simulink model "B2B_MMC"  (R2018b)
settings: Solver=ode8  StartTime=0.0  StopTime=inf  FixedStep=10e-5  RelTol=1e-3
InitFcn:
  | Cd=100e-6;
  | Csm=3.3e-3;
  | L=4e-3;
  | R=0.1;
  | m=1;
  | N=9;
  | Nminus=N-1;
  | 
  | 
  | grid.vll_rms=10e3;
  | grid.f=50;
  | w=2*pi*grid.f;
  | grid.phase=0;
  | grid.va_peak=sqrt(2/3)*grid.vll_rms;
  | 
  | vd_ref=1.05*2*sqrt(2/3)*grid.vll_rms/m; % dc link voltage in pu
  | vsp_max=0.5*m*vd_ref; %phase voltage at phi=0
  | is_max=907;
  | Smax=3*grid.va_peak*is_max/2;
  | 
  | 
  | SCR= 100;  % INPUT SCR of grid at PCC = Ssc_grid/S_rated
  | %Calculated Grid impedance parameters
  | grid.L=grid.va_peak/(w*SCR*is_max); %Calculate Lg out of SRC and neglecting Rg
  | grid.R= w*grid.L/10;        % assume Rg = 10% of Xg [ohm];
  | grid.enable=1;
  | 
  | 
  | 
  | mmc1.load_percent=100;
  | mmc1.load_pf=0.9;
  | 
  | mmc2.load_percent=100;
  | mmc2.load_pf=0.9;
  | 
  | 
  | 
  | mmc1.occ_alpha = 2000;      % INPUT Desired BW output control test converter [rad/s]
  | mmc1.occ_alpha1 = 50;       % INPUT Desired BW of the resonant integrator [rad/s]
  | mmc1.occ_alpha_f = 1000;       % INPUT Desire BW of the VFF [rad/s]
  | 
  | mmc2.occ_alpha = 2000;      % INPUT Desired BW output control test converter [rad/s]
  | mmc2.occ_alpha1 = 50;       % INPUT Desired BW of the resonant integrator [rad/s}
  | mmc2.occ_alpha_f = 1000;       % INPUT Desire BW of the VFF [rad/s
  | 
  | 
  | mmc1.ccc_enable= 1; %INPUT enable ic controller
  | mmc1.ccc_time_enable= 0; %time when circ current control kicks in [s]
  | mmc1.ccc_alpha_cr= 30;  % INPUT BW of LPF for circ current to get the reference (dc value)[rad/s]
  | mmc1.ccc_Ra        = 10;       % INPUT Proportional gain of circ current control (R << Ra < Kp)
  | mmc1.ccc_alpha2 = 200;      % INPUT BW for circulating current test converter  (alpha_c < wgrid)[rad/s]
  | 
  | mmc2.ccc_enable= 1; %INPUT enable ic controller
  | mmc2.ccc_time_enable= 0; %time when circ current control kicks in [s]
  | mmc2.ccc_alpha_cr= 30;  % INPUT BW of LPF for circ current to get the reference (dc value)[rad/s]
  | mmc2.ccc_Ra        = 10;       % INPUT Proportional gain of circ current control (R << Ra < Kp)
  | mmc2.ccc_alpha2 = 200;      % INPUT BW for circulating current test converter  (alpha_c < wgrid)[rad/s]
  | 
  | 
  | mmc1.aec_enable_W= 1; %INPUT enable arm energy controller (Wsum and Wdelta)) at time_W_ctrl
  | ... (+31 lines)
libraries: powerlib x90, powerlib_meascontrol x10, rtlab x1, rtio_opalrt_op5142ex1 x1
(part 2 of 3)

== system B2B_MMC/SM_MMC/MMC1/convertor legs/lower arm a ==
  nla : Inport
  ila : Inport  Port=2
  Controlled Voltage Source : powerlib/Electrical Sources/Controlled Voltage Source  Initialize=on  Source_Type=AC  Amplitude=0  Phase=0  Frequency=0  Measurements=None
  Delay : Delay  DelayLength=1  InitialCondition=0
  Delay1 : Delay  DelayLength=1  InitialCondition=0
  Product : Product
  Product1 : Product
  Voltage Measurement : powerlib/Measurements/Voltage Measurement  PhasorSimulation=off  OutputType=Complex  PSBequivalent=0
  carm : powerlib/Elements/Series RLC Branch  LConnTagsString=__new0  RConnTagsString=__new0  BranchType=C  Resistance=1  Inductance=1e-3  SetiL0=off  InitialCurrent=0  Capacitance=Csm/N  Setx0=on  InitialVoltage=vd_ref  Measurements=None
  icap : powerlib/Electrical Sources/Controlled Current Source  Initialize=on  Source_Type=AC  Amplitude=0  Phase=0  Frequency=0  Measurements=None
  B : PMIOPort  Side=Left
  A : PMIOPort  Port=2  Side=Right
  vc_la : Outport
  wires:
  nla/1 -> Delay/1
  Product/1 -> Controlled Voltage Source/1
  ila/1 -> Delay1/1
  Delay/1 -> Product1/1, Product/2
  Product1/1 -> icap/1
  Voltage Measurement/1 -> vc_la/1, Product/1
  Delay1/1 -> Product1/2
  connections:
  Controlled Voltage Source/LConn1 -- B/RConn1
  Controlled Voltage Source/RConn1 -- A/RConn1
  Voltage Measurement/LConn1 -- carm/LConn1 -- icap/RConn1
  icap/LConn1 -- carm/RConn1 -- Voltage Measurement/LConn2

== system B2B_MMC/SM_MMC/MMC1/convertor legs/lower arm b ==
  nlb : Inport
  ilb : Inport  Port=2
  Controlled Voltage Source : powerlib/Electrical Sources/Controlled Voltage Source  Initialize=on  Source_Type=AC  Amplitude=0  Phase=0  Frequency=0  Measurements=None
  Delay : Delay  DelayLength=1  InitialCondition=0
  Delay1 : Delay  DelayLength=1  InitialCondition=0
  Product : Product
  Product1 : Product
  Voltage Measurement : powerlib/Measurements/Voltage Measurement  PhasorSimulation=off  OutputType=Complex  PSBequivalent=0
  carm : powerlib/Elements/Series RLC Branch  LConnTagsString=__new0  RConnTagsString=__new0  BranchType=C  Resistance=1  Inductance=1e-3  SetiL0=off  InitialCurrent=0  Capacitance=Csm/N  Setx0=on  InitialVoltage=vd_ref  Measurements=None
  icap : powerlib/Electrical Sources/Controlled Current Source  Initialize=on  Source_Type=AC  Amplitude=0  Phase=0  Frequency=0  Measurements=None
  B : PMIOPort  Side=Left
  A : PMIOPort  Port=2  Side=Right
  vc_lb : Outport
  wires:
  nlb/1 -> Delay/1
  Product/1 -> Controlled Voltage Source/1
  ilb/1 -> Delay1/1
  Delay/1 -> Product1/1, Product/2
  Product1/1 -> icap/1
  Voltage Measurement/1 -> vc_lb/1, Product/1
  Delay1/1 -> Product1/2
  connections:
  Controlled Voltage Source/LConn1 -- B/RConn1
  Controlled Voltage Source/RConn1 -- A/RConn1
  Voltage Measurement/LConn1 -- carm/LConn1 -- icap/RConn1
  icap/LConn1 -- carm/RConn1 -- Voltage Measurement/LConn2

== system B2B_MMC/SM_MMC/MMC1/convertor legs/lower arm c ==
  nlc : Inport
  ilc : Inport  Port=2
  Controlled Voltage Source : powerlib/Electrical Sources/Controlled Voltage Source  Initialize=on  Source_Type=AC  Amplitude=0  Phase=0  Frequency=0  Measurements=None
  Delay : Delay  DelayLength=1  InitialCondition=0
  Delay1 : Delay  DelayLength=1  InitialCondition=0
  Product : Product
  Product1 : Product
  Voltage Measurement : powerlib/Measurements/Voltage Measurement  PhasorSimulation=off  OutputType=Complex  PSBequivalent=0
  carm : powerlib/Elements/Series RLC Branch  LConnTagsString=__new0  RConnTagsString=__new0  BranchType=C  Resistance=1  Inductance=1e-3  SetiL0=off  InitialCurrent=0  Capacitance=Csm/N  Setx0=on  InitialVoltage=vd_ref  Measurements=None
  icap : powerlib/Electrical Sources/Controlled Current Source  Initialize=on  Source_Type=AC  Amplitude=0  Phase=0  Frequency=0  Measurements=None
  B : PMIOPort  Side=Left
  A : PMIOPort  Port=2  Side=Right
  vc_lc : Outport
  wires:
  nlc/1 -> Delay/1
  Product/1 -> Controlled Voltage Source/1
  ilc/1 -> Delay1/1
  Delay/1 -> Product1/1, Product/2
  Product1/1 -> icap/1
  Voltage Measurement/1 -> vc_lc/1, Product/1
  Delay1/1 -> Product1/2
  connections:
  Controlled Voltage Source/LConn1 -- B/RConn1
  Controlled Voltage Source/RConn1 -- A/RConn1
  Voltage Measurement/LConn1 -- carm/LConn1 -- icap/RConn1
  icap/LConn1 -- carm/RConn1 -- Voltage Measurement/LConn2

== system B2B_MMC/SM_MMC/MMC1/convertor legs/upper arm a ==
  nua : Inport
  iua : Inport  Port=2
  Controlled Voltage Source : powerlib/Electrical Sources/Controlled Voltage Source  Initialize=on  Source_Type=AC  Amplitude=0  Phase=0  Frequency=0  Measurements=None
  Delay : Delay  DelayLength=1  InitialCondition=0
  Delay1 : Delay  DelayLength=1  InitialCondition=0
  Product : Product
  Product1 : Product
  Voltage Measurement : powerlib/Measurements/Voltage Measurement  PhasorSimulation=off  OutputType=Complex  PSBequivalent=0
  carm : powerlib/Elements/Series RLC Branch  LConnTagsString=__new0  RConnTagsString=__new0  BranchType=C  Resistance=1  Inductance=1e-3  SetiL0=off  InitialCurrent=0  Capacitance=Csm/N  Setx0=on  InitialVoltage=vd_ref  Measurements=None
  icap : powerlib/Electrical Sources/Controlled Current Source  Initialize=on  Source_Type=AC  Amplitude=0  Phase=0  Frequency=0  Measurements=None
  B : PMIOPort  Side=Left
  A : PMIOPort  Port=2  Side=Right
  vc_ua : Outport
  wires:
  nua/1 -> Delay/1
  Product/1 -> Controlled Voltage Source/1
  iua/1 -> Delay1/1
  Delay/1 -> Product1/1, Product/2
  Product1/1 -> icap/1
  Voltage Measurement/1 -> vc_ua/1, Product/1
  Delay1/1 -> Product1/2
  connections:
  Controlled Voltage Source/LConn1 -- B/RConn1
  Controlled Voltage Source/RConn1 -- A/RConn1
  carm/LConn1 -- icap/RConn1 -- Voltage Measurement/LConn1
  carm/RConn1 -- Voltage Measurement/LConn2 -- icap/LConn1

== system B2B_MMC/SM_MMC/MMC1/convertor legs/upper arm b ==
  nub : Inport
  iub : Inport  Port=2
  Controlled Voltage Source : powerlib/Electrical Sources/Controlled Voltage Source  Initialize=on  Source_Type=AC  Amplitude=0  Phase=0  Frequency=0  Measurements=None
  Delay : Delay  DelayLength=1  InitialCondition=0
  Delay1 : Delay  DelayLength=1  InitialCondition=0
  Product : Product
  Product1 : Product
  Voltage Measurement : powerlib/Measurements/Voltage Measurement  PhasorSimulation=off  OutputType=Complex  PSBequivalent=0
  carm : powerlib/Elements/Series RLC Branch  LConnTagsString=__new0  RConnTagsString=__new0  BranchType=C  Resistance=1  Inductance=1e-3  SetiL0=off  InitialCurrent=0  Capacitance=Csm/N  Setx0=on  InitialVoltage=vd_ref  Measurements=None
  icap : powerlib/Electrical Sources/Controlled Current Source  Initialize=on  Source_Type=AC  Amplitude=0  Phase=0  Frequency=0  Measurements=None
  B : PMIOPort  Side=Left
  A : PMIOPort  Port=2  Side=Right
  vc_ub : Outport
  wires:
  nub/1 -> Delay/1
  Product/1 -> Controlled Voltage Source/1
  iub/1 -> Delay1/1
  Delay/1 -> Product1/1, Product/2
  Product1/1 -> icap/1
  Voltage Measurement/1 -> vc_ub/1, Product/1
  Delay1/1 -> Product1/2
  connections:
  Controlled Voltage Source/LConn1 -- B/RConn1
  Controlled Voltage Source/RConn1 -- A/RConn1
  Voltage Measurement/LConn1 -- carm/LConn1 -- icap/RConn1
  icap/LConn1 -- carm/RConn1 -- Voltage Measurement/LConn2

== system B2B_MMC/SM_MMC/MMC1/convertor legs/upper arm c ==
  nuc : Inport
  iuc : Inport  Port=2
  Controlled Voltage Source : powerlib/Electrical Sources/Controlled Voltage Source  Initialize=on  Source_Type=AC  Amplitude=0  Phase=0  Frequency=0  Measurements=None
  Delay : Delay  DelayLength=1  InitialCondition=0
  Delay1 : Delay  DelayLength=1  InitialCondition=0
  Product : Product
  Product1 : Product
  Voltage Measurement : powerlib/Measurements/Voltage Measurement  PhasorSimulation=off  OutputType=Complex  PSBequivalent=0
  carm : powerlib/Elements/Series RLC Branch  LConnTagsString=__new0  RConnTagsString=__new0  BranchType=C  Resistance=1  Inductance=1e-3  SetiL0=off  InitialCurrent=0  Capacitance=Csm/N  Setx0=on  InitialVoltage=vd_ref  Measurements=None
  icap : powerlib/Electrical Sources/Controlled Current Source  Initialize=on  Source_Type=AC  Amplitude=0  Phase=0  Frequency=0  Measurements=None
  B : PMIOPort  Side=Left
  A : PMIOPort  Port=2  Side=Right
  vc_uc : Outport
  wires:
  nuc/1 -> Delay/1
  Product/1 -> Controlled Voltage Source/1
  iuc/1 -> Delay1/1
  Delay/1 -> Product1/1, Product/2
  Product1/1 -> icap/1
  Voltage Measurement/1 -> vc_uc/1, Product/1
  Delay1/1 -> Product1/2
  connections:
  Controlled Voltage Source/LConn1 -- B/RConn1
  Controlled Voltage Source/RConn1 -- A/RConn1
  Voltage Measurement/LConn1 -- carm/LConn1 -- icap/RConn1
  icap/LConn1 -- carm/RConn1 -- Voltage Measurement/LConn2

== system B2B_MMC/SM_MMC/MMC2/Control Box MMC2/Capacitor Voltages ==
  Mux : Mux  Inputs=2
  Mux2 : Mux  Inputs=2
  Mux3 : Mux  Inputs=2
  Sum of Elements{,1..5} (6 alike) : Sum  Inputs=+
  sum_vca_ul : Outport
  sum_vcb_ul : Outport  Port=2
  sum_vcc_ul : Outport  Port=3
  wires:
  [vc_ua] -> Sum of Elements/1
  [vc_la] -> Sum of Elements1/1
  [vc_uc] -> Sum of Elements4/1
  [vc_lc] -> Sum of Elements5/1
  [vc_lb] -> Sum of Elements3/1
  [vc_ub] -> Sum of Elements2/1
  Mux2/1 -> sum_vcb_ul/1
  Sum of Elements4/1 -> Mux3/1
  Sum of Elements/1 -> Mux/1
  Sum of Elements3/1 -> Mux2/2
  Sum of Elements2/1 -> Mux2/1
  Mux/1 -> sum_vca_ul/1
  Mux3/1 -> sum_vcc_ul/1
  Sum of Elements1/1 -> Mux/2
  Sum of Elements5/1 -> Mux3/2

== system B2B_MMC/SM_MMC/MMC2/Control Box MMC2/Controllers ==
  is* : Inport
  vpcc_ab : Inport  Port=2
  is_ab : Inport  Port=3
  ic : Inport  Port=4
  Circulating Current and Arm Energy Controller : Subsystem
  PR Output Current Controller : Subsystem
  vs* : Outport
  vc* : Outport  Port=2
  wires:
  Circulating Current and Arm Energy Controller/1(vc*) -> vc*/1
  PR Output Current Controller/1(vs*) -> vs*/1
  is*/1 -> PR Output Current Controller/1(isAB*)
  ic/1 -> Circulating Current and Arm Energy Controller/1(Ic)
  is_ab/1 -> PR Output Current Controller/2(is_ab)
  vpcc_ab/1 -> PR Output Current Controller/3(vpcc_ab)

== system B2B_MMC/SM_MMC/MMC2/Control Box MMC2/Current Transforms ==
  Gain : Gain  Gain=0.5
  Sum : Sum  Inputs=|+-
  Sum1 : Sum  Inputs=|++
  is : Outport
  ic : Outport  Port=2
  wires:
  Gain/1 -> ic/1
  Sum1/1 -> Gain/1
  [iu] -> Sum1/1, Sum/1
  Sum/1 -> is/1
  [il] -> Sum/2, Sum1/2

== system B2B_MMC/SM_MMC/MMC2/Control Box MMC2/Insertion Indices (Direct Voltage Control) ==
  note: vs_ref
  note: vd/2
  note: vl_ref
  note: vu_ref
  note: vd/2
  note: vs_ref
  vs* : Inport
  vc* : Inport  Port=2
  Divide : Product  Inputs=*/
  Divide1 : Product  Inputs=*/
  Saturation1 : Saturate  UpperLimit=1  LowerLimit=0
  Saturation2 : Saturate  UpperLimit=1  LowerLimit=0
  Subsystem : Subsystem  Commented=on
  Sum1 : Sum  Inputs=|+-
  Sum2 : Sum  Inputs=|++
  vd : Constant  Value=vd_ref
  nu : Outport
  nl : Outport  Port=2
  wires:
  vc*/1 -> Sum2/1, Sum1/1
  Sum1/1 -> Divide/1
  vd/1 -> Divide/2, Divide1/2
  vs*/1 -> Sum1/2, Sum2/2
  Sum2/1 -> Divide1/1
  Divide/1 -> Saturation1/1
  Divide1/1 -> Saturation2/1
  Saturation1/1 -> nu/1
  Saturation2/1 -> nl/1

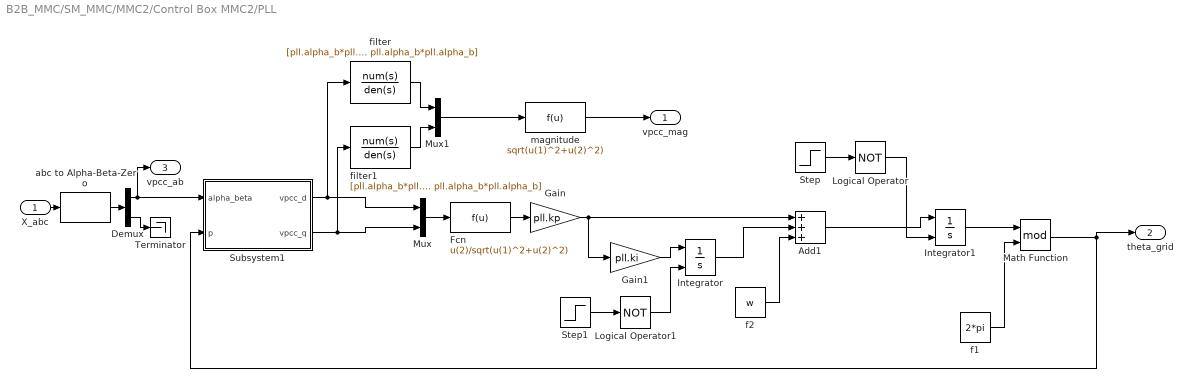
== system B2B_MMC/SM_MMC/MMC2/Control Box MMC2/PLL ==
  X_abc : Inport
  Add1 : Sum  Inputs=+++
  Demux : Demux  Outputs=2
  Fcn : Fcn  Expr=u(2)/sqrt(u(1)^2+u(2)^2)
  Gain : Gain  Gain=pll.kp
  Gain1 : Gain  Gain=pll.ki
  Integrator : Integrator  ExternalReset=level
  Integrator1 : Integrator  ExternalReset=level  InitialCondition=w
  Logical Operator : Logic  Operator=NOT  AllPortsSameDT=off  OutDataTypeStr=boolean
  Logical Operator1 : Logic  Operator=NOT  AllPortsSameDT=off  OutDataTypeStr=boolean
  Math Function : Math  Operator=mod  SaturateOnIntegerOverflow=on
  Mux : Mux  Inputs=2
  Mux1 : Mux  Inputs=2
  Step : Step  Time=1e-6  After=grid.enable  SampleTime=0
  Step1 : Step  Time=1e-6  After=grid.enable  SampleTime=0
  Subsystem1 : Subsystem
  Terminator : Terminator
  abc to Alpha-Beta-Zero : powerlib_meascontrol/Transformations/abc to Alpha-Beta-Zero
      settings: SourceProductName=Simscape Power Systems
  f1 : Constant  Value=2*pi
  f2 : Constant  Value=w
  filter : TransferFcn  Numerator=[pll.alpha_b*pll.alpha_b]  Denominator=[1 sqrt(2)*pll.alpha_b pll.alpha_b*pll.alpha_b]
  filter1 : TransferFcn  Numerator=[pll.alpha_b*pll.alpha_b]  Denominator=[1 sqrt(2)*pll.alpha_b pll.alpha_b*pll.alpha_b]
  magnitude : Fcn  Expr=sqrt(u(1)^2+u(2)^2)
  vpcc_mag : Outport
  theta_grid : Outport  Port=2
  vpcc_ab : Outport  Port=3
  wires:
  Add1/1 -> Integrator1/1
  Fcn/1 -> Gain/1
  Gain1/1 -> Integrator/1
  Gain/1 -> Add1/1, Gain1/1
  Integrator/1 -> Add1/2
  f2/1 -> Add1/3
  Integrator1/1 -> Math Function/1
  f1/1 -> Math Function/2
  Math Function/1 -> theta_grid/1, Subsystem1/2(p)
  Logical Operator1/1 -> Integrator/2
  Logical Operator/1 -> Integrator1/2
  Step1/1 -> Logical Operator1/1
  Demux/1 -> Subsystem1/1(alpha_beta), vpcc_ab/1
  abc to Alpha-Beta-Zero/1 -> Demux/1
  X_abc/1 -> abc to Alpha-Beta-Zero/1
  Demux/2 -> Terminator/1
  Mux/1 -> Fcn/1
  magnitude/1 -> vpcc_mag/1
  Subsystem1/2(vpcc_q) -> filter1/1, Mux/2
  Subsystem1/1(vpcc_d) -> Mux/1, filter/1
  filter/1 -> Mux1/1
  filter1/1 -> Mux1/2
  Mux1/1 -> magnitude/1
  Step/1 -> Logical Operator/1

== system B2B_MMC/SM_MMC/MMC2/Control Box MMC2/Reference Powers ==
  Product : Product
  Product1 : Product
  Product2 : Product
  Trigonometric Function : Trigonometry  Operator=cos
  Trigonometric Function1 : Trigonometry
  percentage loading : Constant  Value=load.percent
  percentage loading1 : Constant  Value=load.phi
  rated converter apparent power : Constant  Value=Smax
  p* : Outport
  q* : Outport  Port=2
  wires:
  rated converter apparent power/1 -> Product/1
  percentage loading/1 -> Product/2
  percentage loading1/1 -> Trigonometric Function/1, Trigonometric Function1/1
  Trigonometric Function/1 -> Product1/1
  Product/1 -> Product2/1, Product1/2
  Trigonometric Function1/1 -> Product2/2
  Product2/1 -> q*/1
  Product1/1 -> p*/1

== system B2B_MMC/SM_MMC/MMC2/Control Box MMC2/Subsystem ==
  vpcc : Inport
  is_meas : Inport  Port=2
  Demux{,1..3} (4 alike) : Demux  Outputs=3
  Fcn : Fcn  Expr=(u(1)*u(4)) + (u(2)*u(5)) + (u(3)*u(6))
  Fcn1 : Fcn  Expr="( (u(1)-u(2))*u(6) +  (u(3)-u(1))*u(5)  + (u(2)-u(3))*u(4) )/sqrt(3)"
  Mux1 : Mux  Inputs=2
  Mux2 : Mux  Inputs=2
  Mux3 : Mux  Inputs=6
  Transfer Fcn : TransferFcn  Numerator=[2*pi*5]  Denominator=[1 2*pi*5]
  Transfer Fcn1 : TransferFcn  Numerator=[2*pi*5]  Denominator=[1 2*pi*5]
  vs : Outport
  is : Outport  Port=2
  meas_p : Outport  Port=3
  meas_q : Outport  Port=4
  wires:
  Demux/1 -> Mux3/1, Mux2/1
  Demux3/1 -> Mux2/2
  [vsref_abc] -> Demux3/1
  Demux2/1 -> Mux1/2
  Demux1/1 -> Mux3/4, Mux1/1
  Mux2/1 -> vs/1
  vpcc/1 -> Demux/1
  is_meas/1 -> Demux1/1
  Mux1/1 -> is/1
  [isref_abc] -> Demux2/1
  Fcn/1 -> Transfer Fcn/1
  Demux/2 -> Mux3/2
  Demux/3 -> Mux3/3
  Mux3/1 -> Fcn1/1, Fcn/1
  Demux1/2 -> Mux3/5
  Demux1/3 -> Mux3/6
  Transfer Fcn/1 -> meas_p/1
  Transfer Fcn1/1 -> meas_q/1
  Fcn1/1 -> Transfer Fcn1/1

== system B2B_MMC/SM_MMC/MMC2/Control Box MMC2/Transform1 ==
  is : Inport
  Demux : Demux  Outputs=2
  Terminator : Terminator
  abc to Alpha-Beta-Zero : powerlib_meascontrol/Transformations/abc to Alpha-Beta-Zero
      settings: SourceProductName=Simscape Power Systems
  is_ab : Outport
  wires:
  is/1 -> abc to Alpha-Beta-Zero/1
  abc to Alpha-Beta-Zero/1 -> Demux/1
  Demux/1 -> is_ab/1
  Demux/2 -> Terminator/1

== system B2B_MMC/SM_MMC/MMC2/Control Box MMC2/is_ref ==
  vd : Inport
  p* : Inport  Port=2
  q* : Inport  Port=3
  vpll_mag : Inport  Port=4
  theta : Inport  Port=5
  Add1 : Sum  Inputs=+-
  Alpha-Beta-Zero to abc : powerlib_meascontrol/Transformations/Alpha-Beta-Zero to abc
      settings: SourceProductName=Simscape Power Systems  SourceProductBaseCode=PS
  Constant : Constant  Value=0
  Constant1 : Constant  Value=cvdc.enable
  Demux : Demux  Outputs=2
  Divide : Product  Inputs=*/
  Divide1 : Product  Inputs=/*
  Divide2 : Product  Inputs=**
  Gain : Gain  Gain=2/3
  Gain1 : Gain  Gain=-2/3
  Gain2 : Gain  Gain=3/2
  Mux : Mux  Inputs=3
  Saturation1 : Saturate  UpperLimit=is_max  LowerLimit=-is_max
  Saturation2 : Saturate  UpperLimit=is_max  LowerLimit=-is_max
  Saturation3 : Saturate  UpperLimit=1e9  LowerLimit=1e-6
  Switch : Switch  Criteria=u2 > Threshold
  Terminator : Terminator
  dc link voltage control : Subsystem
  dq0 to Alpha-Beta-Zero : powerlib_meascontrol/Transformations/dq0 to Alpha-Beta-Zero  Alignment=Aligned with phase A axis
      settings: SourceProductName=Simscape Power Systems  SourceProductBaseCode=PS
  is_abc : Outport
  is_ab* : Outport  Port=2
  wires:
  q*/1 -> Gain1/1
  Gain/1 -> Divide/1
  Saturation3/1 -> Divide/2, Divide2/2, Divide1/1
  Gain1/1 -> Divide1/2
  Constant/1 -> Mux/3
  Mux/1 -> dq0 to Alpha-Beta-Zero/1
  dq0 to Alpha-Beta-Zero/1 -> Alpha-Beta-Zero to abc/1, Demux/1
  Demux/2 -> Terminator/1
  Demux/1 -> is_ab*/1
  theta/1 -> dq0 to Alpha-Beta-Zero/2
  Divide/1 -> Add1/2, Saturation1/1
  Saturation1/1 -> Add1/1, Mux/1
  Divide1/1 -> Saturation2/1
  Saturation2/1 -> Mux/2
  vpll_mag/1 -> Saturation3/1
  Alpha-Beta-Zero to abc/1 -> is_abc/1
  vd/1 -> dc link voltage control/2(vd)
  Add1/1 -> Divide2/1
  Divide2/1 -> Gain2/1
  Gain2/1 -> dc link voltage control/1(antiwp)
  Switch/1 -> Gain/1
  dc link voltage control/1(p*) -> Switch/1
  p*/1 -> Switch/3
  Constant1/1 -> Switch/2

== system B2B_MMC/SM_MMC/MMC2/convertor legs/lower arm a ==
  nla : Inport
  ila : Inport  Port=2
  Controlled Voltage Source : powerlib/Electrical Sources/Controlled Voltage Source  Initialize=on  Source_Type=AC  Amplitude=0  Phase=0  Frequency=0  Measurements=None
  Delay : Delay  DelayLength=1  InitialCondition=0
  Delay1 : Delay  DelayLength=1  InitialCondition=0
  Product : Product
  Product1 : Product
  Voltage Measurement : powerlib/Measurements/Voltage Measurement  PhasorSimulation=off  OutputType=Complex  PSBequivalent=0
  carm : powerlib/Elements/Series RLC Branch  LConnTagsString=__new0  RConnTagsString=__new0  BranchType=C  Resistance=1  Inductance=1e-3  SetiL0=off  InitialCurrent=0  Capacitance=Csm/N  Setx0=on  InitialVoltage=vd_ref  Measurements=None
  icap : powerlib/Electrical Sources/Controlled Current Source  Initialize=on  Source_Type=AC  Amplitude=0  Phase=0  Frequency=0  Measurements=None
  B : PMIOPort  Side=Left
  A : PMIOPort  Port=2  Side=Right
  vc_la : Outport
  wires:
  nla/1 -> Delay/1
  Product/1 -> Controlled Voltage Source/1
  ila/1 -> Delay1/1
  Delay/1 -> Product1/1, Product/2
  Product1/1 -> icap/1
  Voltage Measurement/1 -> vc_la/1, Product/1
  Delay1/1 -> Product1/2
  connections:
  Controlled Voltage Source/LConn1 -- B/RConn1
  Controlled Voltage Source/RConn1 -- A/RConn1
  Voltage Measurement/LConn1 -- carm/LConn1 -- icap/RConn1
  icap/LConn1 -- carm/RConn1 -- Voltage Measurement/LConn2

== system B2B_MMC/SM_MMC/MMC2/convertor legs/lower arm b ==
  nlb : Inport
  ilb : Inport  Port=2
  Controlled Voltage Source : powerlib/Electrical Sources/Controlled Voltage Source  Initialize=on  Source_Type=AC  Amplitude=0  Phase=0  Frequency=0  Measurements=None
  Delay : Delay  DelayLength=1  InitialCondition=0
  Delay1 : Delay  DelayLength=1  InitialCondition=0
  Product : Product
  Product1 : Product
  Voltage Measurement : powerlib/Measurements/Voltage Measurement  PhasorSimulation=off  OutputType=Complex  PSBequivalent=0
  carm : powerlib/Elements/Series RLC Branch  LConnTagsString=__new0  RConnTagsString=__new0  BranchType=C  Resistance=1  Inductance=1e-3  SetiL0=off  InitialCurrent=0  Capacitance=Csm/N  Setx0=on  InitialVoltage=vd_ref  Measurements=None
  icap : powerlib/Electrical Sources/Controlled Current Source  Initialize=on  Source_Type=AC  Amplitude=0  Phase=0  Frequency=0  Measurements=None
  B : PMIOPort  Side=Left
  A : PMIOPort  Port=2  Side=Right
  vc_lb : Outport
  wires:
  nlb/1 -> Delay/1
  Product/1 -> Controlled Voltage Source/1
  ilb/1 -> Delay1/1
  Delay/1 -> Product1/1, Product/2
  Product1/1 -> icap/1
  Voltage Measurement/1 -> vc_lb/1, Product/1
  Delay1/1 -> Product1/2
  connections:
  Controlled Voltage Source/LConn1 -- B/RConn1
  Controlled Voltage Source/RConn1 -- A/RConn1
  Voltage Measurement/LConn1 -- carm/LConn1 -- icap/RConn1
  icap/LConn1 -- carm/RConn1 -- Voltage Measurement/LConn2

== system B2B_MMC/SM_MMC/MMC2/convertor legs/lower arm c ==
  nlc : Inport
  ilc : Inport  Port=2
  Controlled Voltage Source : powerlib/Electrical Sources/Controlled Voltage Source  Initialize=on  Source_Type=AC  Amplitude=0  Phase=0  Frequency=0  Measurements=None
  Delay : Delay  DelayLength=1  InitialCondition=0
  Delay1 : Delay  DelayLength=1  InitialCondition=0
  Product : Product
  Product1 : Product
  Voltage Measurement : powerlib/Measurements/Voltage Measurement  PhasorSimulation=off  OutputType=Complex  PSBequivalent=0
  carm : powerlib/Elements/Series RLC Branch  LConnTagsString=__new0  RConnTagsString=__new0  BranchType=C  Resistance=1  Inductance=1e-3  SetiL0=off  InitialCurrent=0  Capacitance=Csm/N  Setx0=on  InitialVoltage=vd_ref  Measurements=None
  icap : powerlib/Electrical Sources/Controlled Current Source  Initialize=on  Source_Type=AC  Amplitude=0  Phase=0  Frequency=0  Measurements=None
  B : PMIOPort  Side=Left
  A : PMIOPort  Port=2  Side=Right
  vc_lc : Outport
  wires:
  nlc/1 -> Delay/1
  Product/1 -> Controlled Voltage Source/1
  ilc/1 -> Delay1/1
  Delay/1 -> Product1/1, Product/2
  Product1/1 -> icap/1
  Voltage Measurement/1 -> vc_lc/1, Product/1
  Delay1/1 -> Product1/2
  connections:
  Controlled Voltage Source/LConn1 -- B/RConn1
  Controlled Voltage Source/RConn1 -- A/RConn1
  Voltage Measurement/LConn1 -- carm/LConn1 -- icap/RConn1
  icap/LConn1 -- carm/RConn1 -- Voltage Measurement/LConn2

== system B2B_MMC/SM_MMC/MMC2/convertor legs/upper arm a ==
  nua : Inport
  iua : Inport  Port=2
  Controlled Voltage Source : powerlib/Electrical Sources/Controlled Voltage Source  Initialize=on  Source_Type=AC  Amplitude=0  Phase=0  Frequency=0  Measurements=None
  Delay : Delay  DelayLength=1  InitialCondition=0
  Delay1 : Delay  DelayLength=1  InitialCondition=0
  Delay2 : Delay  DelayLength=1  InitialCondition=0
  Product : Product
  Product1 : Product
  Voltage Measurement : powerlib/Measurements/Voltage Measurement  PhasorSimulation=off  OutputType=Complex  PSBequivalent=0
  carm : powerlib/Elements/Series RLC Branch  LConnTagsString=__new0  RConnTagsString=__new0  BranchType=C  Resistance=1  Inductance=1e-3  SetiL0=off  InitialCurrent=0  Capacitance=Csm/N  Setx0=on  InitialVoltage=vd_ref  Measurements=None
  icap : powerlib/Electrical Sources/Controlled Current Source  Initialize=on  Source_Type=AC  Amplitude=0  Phase=0  Frequency=0  Measurements=None
  B : PMIOPort  Side=Left
  A : PMIOPort  Port=2  Side=Right
  vc_ua : Outport
  wires:
  nua/1 -> Delay/1
  Product/1 -> Controlled Voltage Source/1
  iua/1 -> Delay2/1
  Delay/1 -> Product1/1, Product/2
  Product1/1 -> Delay1/1
  Voltage Measurement/1 -> vc_ua/1, Product/1
  Delay1/1 -> icap/1
  Delay2/1 -> Product1/2
  connections:
  Controlled Voltage Source/LConn1 -- B/RConn1
  Controlled Voltage Source/RConn1 -- A/RConn1
  carm/LConn1 -- icap/RConn1 -- Voltage Measurement/LConn1
  carm/RConn1 -- Voltage Measurement/LConn2 -- icap/LConn1

== system B2B_MMC/SM_MMC/MMC2/convertor legs/upper arm b ==
  nub : Inport
  iub : Inport  Port=2
  Controlled Voltage Source : powerlib/Electrical Sources/Controlled Voltage Source  Initialize=on  Source_Type=AC  Amplitude=0  Phase=0  Frequency=0  Measurements=None
  Delay : Delay  DelayLength=1  InitialCondition=0
  Delay1 : Delay  DelayLength=1  InitialCondition=0
  Product : Product
  Product1 : Product
  Voltage Measurement : powerlib/Measurements/Voltage Measurement  PhasorSimulation=off  OutputType=Complex  PSBequivalent=0
  carm : powerlib/Elements/Series RLC Branch  LConnTagsString=__new0  RConnTagsString=__new0  BranchType=C  Resistance=1  Inductance=1e-3  SetiL0=off  InitialCurrent=0  Capacitance=Csm/N  Setx0=on  InitialVoltage=vd_ref  Measurements=None
  icap : powerlib/Electrical Sources/Controlled Current Source  Initialize=on  Source_Type=AC  Amplitude=0  Phase=0  Frequency=0  Measurements=None
  B : PMIOPort  Side=Left
  A : PMIOPort  Port=2  Side=Right
  vc_ub : Outport
  wires:
  nub/1 -> Delay/1
  Product/1 -> Controlled Voltage Source/1
  iub/1 -> Delay1/1
  Delay/1 -> Product1/1, Product/2
  Product1/1 -> icap/1
  Voltage Measurement/1 -> vc_ub/1, Product/1
  Delay1/1 -> Product1/2
  connections:
  Controlled Voltage Source/LConn1 -- B/RConn1
  Controlled Voltage Source/RConn1 -- A/RConn1
  Voltage Measurement/LConn1 -- carm/LConn1 -- icap/RConn1
  icap/LConn1 -- carm/RConn1 -- Voltage Measurement/LConn2

== system B2B_MMC/SM_MMC/MMC2/convertor legs/upper arm c ==
  nuc : Inport
  iuc : Inport  Port=2
  Controlled Voltage Source : powerlib/Electrical Sources/Controlled Voltage Source  Initialize=on  Source_Type=AC  Amplitude=0  Phase=0  Frequency=0  Measurements=None
  Delay : Delay  DelayLength=1  InitialCondition=0
  Delay1 : Delay  DelayLength=1  InitialCondition=0
  Product : Product
  Product1 : Product
  Voltage Measurement : powerlib/Measurements/Voltage Measurement  PhasorSimulation=off  OutputType=Complex  PSBequivalent=0
  carm : powerlib/Elements/Series RLC Branch  LConnTagsString=__new0  RConnTagsString=__new0  BranchType=C  Resistance=1  Inductance=1e-3  SetiL0=off  InitialCurrent=0  Capacitance=Csm/N  Setx0=on  InitialVoltage=vd_ref  Measurements=None
  icap : powerlib/Electrical Sources/Controlled Current Source  Initialize=on  Source_Type=AC  Amplitude=0  Phase=0  Frequency=0  Measurements=None
  B : PMIOPort  Side=Left
  A : PMIOPort  Port=2  Side=Right
  vc_uc : Outport
  wires:
  nuc/1 -> Delay/1
  Product/1 -> Controlled Voltage Source/1
  iuc/1 -> Delay1/1
  Delay/1 -> Product1/1, Product/2
  Product1/1 -> icap/1
  Voltage Measurement/1 -> vc_uc/1, Product/1
  Delay1/1 -> Product1/2
  connections:
  Controlled Voltage Source/LConn1 -- B/RConn1
  Controlled Voltage Source/RConn1 -- A/RConn1
  Voltage Measurement/LConn1 -- carm/LConn1 -- icap/RConn1
  icap/LConn1 -- carm/RConn1 -- Voltage Measurement/LConn2

== system B2B_MMC/SM_MMC/MMC1/Control Box MMC1/Controllers/Circulating Current and Arm Energy Controller ==
  Ic : Inport
  BW : Subsystem
  Constant2 : Constant  Value=vd_ref/2
  Constant4 : Constant  Value=ccc.alpha_cr  SampleTime=-1
  Divide : Product  Inputs=**
  Enable Icirc controller Time: time_enable_int_ctrl : Step  Time=ccc.time_enable_int_ctrl  After=ccc.enable_int_ctrl  SampleTime=0
  Goto Tag Visibility : GotoTagVisibility  GotoTag=IC_RST2
  Goto Tag Visibility1 : GotoTagVisibility  GotoTag=enable_W_ctrl2
  Logical Operator : Logic  Operator=NOT  AllPortsSameDT=off  OutDataTypeStr=boolean
  Sum1 : Sum  Inputs=|+-
  Sum3 : Sum  Inputs=|++
  Sum4 : Sum  Inputs=|++
  "arm energy controller " : Subsystem
  ic controller : Subsystem
  vc* : Outport
  tag scope: IC_RST2=scoped, enable_W_ctrl2=scoped
  wires:
  [IC_RST2] -> BW/3(RST)
  Ic/1 -> BW/1(In), Sum1/2
  Enable Icirc controller Time: time_enable_int_ctrl/1 -> Divide/2, Logical Operator/1
  Sum3/1 -> ic controller/1(ic*)
  Divide/1 -> Sum4/1
  Logical Operator/1 -> [IC_RST2]
  Sum1/1 -> Sum3/1
  BW/1(Out) -> Sum1/1
  Constant4/1 -> BW/2(alpha)
  Sum4/1 -> vc*/1
  ic controller/1("vc* ") -> Divide/1
  Constant2/1 -> Sum4/2
  "arm energy controller "/1(delta_i_a) -> [enable_W_ctrl2], Sum3/2

== system B2B_MMC/SM_MMC/MMC1/Control Box MMC1/Controllers/PR Output Current Controller ==
  isAB* : Inport
  is_ab : Inport  Port=2
  vpcc_ab : Inport  Port=3
  Alpha-Beta-Zero to abc : powerlib_meascontrol/Transformations/Alpha-Beta-Zero to abc
      settings: SourceProductName=Simscape Power Systems  SourceProductBaseCode=PS
  Constant : Constant  Value=0  SampleTime=-1
  Mux : Mux  Inputs=2
  Subsystem : Subsystem
  vs* : Outport
  wires:
  Subsystem/1(vsAB_ref) -> Mux/1
  vpcc_ab/1 -> Subsystem/1(FF)
  Mux/1 -> Alpha-Beta-Zero to abc/1
  Constant/1 -> Mux/2
  isAB*/1 -> Subsystem/2(Ref)
  is_ab/1 -> Subsystem/3(FB)
  Alpha-Beta-Zero to abc/1 -> vs*/1

== system B2B_MMC/SM_MMC/MMC1/Control Box MMC1/Insertion Indices (Direct Voltage Control)/Subsystem ==
  Gain1 : Gain  Gain=0.5
  Gain2 : Gain  Gain=m
  Product1 : Product
  Sine Wave1 : Sin  Frequency=w  Phase=[0 2*pi/3 -2*pi/3]  SampleTime=0
  vd1 : Constant  Value=vd_ref
  vs_ref : Outport
  wires:
  vd1/1 -> Gain1/1
  Product1/1 -> vs_ref/1
  Gain1/1 -> Gain2/1
  Gain2/1 -> Product1/1
  Sine Wave1/1 -> Product1/2

== system B2B_MMC/SM_MMC/MMC1/Control Box MMC1/PLL/Subsystem1 ==
  alpha_beta : Inport
  p : Inport  Port=2
  Demux : Demux  Outputs=2
  Gain : Gain
  Product{1..4} (4 alike) : Product
  Sum : Sum  Inputs=|++
  Sum1 : Sum  Inputs=|-+
  Trigonometric Function : Trigonometry  Operator=cos
  Trigonometric Function1 : Trigonometry
  vpcc_d : Outport
  vpcc_q : Outport  Port=2
  wires:
  Trigonometric Function/1 -> Product4/2, Product3/2
  Demux/1 -> Product2/2, Product3/1
  Demux/2 -> Product4/1, Product1/1
  Trigonometric Function1/1 -> Product2/1, Product1/2
  Product1/1 -> Sum/2
  Product2/1 -> Sum1/1
  Product3/1 -> Sum/1
  Product4/1 -> Sum1/2
  alpha_beta/1 -> Demux/1
  p/1 -> Gain/1
  Gain/1 -> Trigonometric Function1/1, Trigonometric Function/1
  Sum1/1 -> vpcc_q/1
  Sum/1 -> vpcc_d/1

== system B2B_MMC/SM_MMC/MMC1/Control Box MMC1/is_ref/dc link voltage control ==
  antiwp : Inport
  vd : Inport  Port=2
  Add : Sum  Inputs=-+
  Add1 : Sum
  Add2 : Sum
  Constant1 : Constant  Value=vd_ref^2
  Divide2 : Product  Inputs=**
  Gain1 : Gain  Gain=cvdc.alpha_id
  Gain2 : Gain  Gain=cvdc.alpha_d*0.5*(Cd+((2*3*Csm)/N))
  Gain3 : Gain  Gain=1/(cvdc.alpha_d*0.5*(Cd+((2*3*Csm)/N)))
  Integrator : Integrator
  filter : TransferFcn  Numerator=[pll.alpha_b*pll.alpha_b]  Denominator=[1 sqrt(2)*pll.alpha_b pll.alpha_b*pll.alpha_b]
  p* : Outport
  wires:
  vd/1 -> filter/1
  filter/1 -> Divide2/2, Divide2/1
  Constant1/1 -> Add/1
  Gain2/1 -> Add2/1, Add1/1
  Add/1 -> Gain2/1
  Divide2/1 -> Add/2
  Add1/1 -> Integrator/1
  Integrator/1 -> Gain1/1
  antiwp/1 -> Gain3/1
  Gain1/1 -> Add2/2
  Add2/1 -> p*/1
  Gain3/1 -> Add1/2

== system B2B_MMC/SM_MMC/MMC2/Control Box MMC2/Controllers/Circulating Current and Arm Energy Controller ==
  Ic : Inport
  BW : Subsystem
  Constant2 : Constant  Value=vd_ref/2
  Constant4 : Constant  Value=ccc.alpha_cr  SampleTime=-1
  Divide : Product  Inputs=**
  Enable Icirc controller Time: time_enable_int_ctrl : Step  Time=ccc.time_enable_int_ctrl  After=ccc.enable_int_ctrl  SampleTime=0
  Goto Tag Visibility : GotoTagVisibility  GotoTag=IC_RST2
  Goto Tag Visibility1 : GotoTagVisibility  GotoTag=enable_W_ctrl2
  Logical Operator : Logic  Operator=NOT  AllPortsSameDT=off  OutDataTypeStr=boolean
  Sum1 : Sum  Inputs=|+-
  Sum3 : Sum  Inputs=|++
  Sum4 : Sum  Inputs=|++
  "arm energy controller " : Subsystem
  ic controller : Subsystem
  vc* : Outport
  tag scope: IC_RST2=scoped, enable_W_ctrl2=scoped
  wires:
  [IC_RST2] -> BW/3(RST)
  Ic/1 -> BW/1(In), Sum1/2
  Enable Icirc controller Time: time_enable_int_ctrl/1 -> Divide/2, Logical Operator/1
  Sum3/1 -> ic controller/1(ic*)
  Divide/1 -> Sum4/1
  Logical Operator/1 -> [IC_RST2]
  Sum1/1 -> Sum3/1
  BW/1(Out) -> Sum1/1
  Constant4/1 -> BW/2(alpha)
  Sum4/1 -> vc*/1
  ic controller/1("vc* ") -> Divide/1
  Constant2/1 -> Sum4/2
  "arm energy controller "/1(delta_i_a) -> [enable_W_ctrl2], Sum3/2

== system B2B_MMC/SM_MMC/MMC2/Control Box MMC2/Controllers/PR Output Current Controller ==
  isAB* : Inport
  is_ab : Inport  Port=2
  vpcc_ab : Inport  Port=3
  Alpha-Beta-Zero to abc : powerlib_meascontrol/Transformations/Alpha-Beta-Zero to abc
      settings: SourceProductName=Simscape Power Systems  SourceProductBaseCode=PS
  Constant : Constant  Value=0  SampleTime=-1
  Mux : Mux  Inputs=2
  Subsystem : Subsystem
  vs* : Outport
  wires:
  Subsystem/1(vsAB_ref) -> Mux/1
  vpcc_ab/1 -> Subsystem/1(FF)
  Mux/1 -> Alpha-Beta-Zero to abc/1
  Constant/1 -> Mux/2
  isAB*/1 -> Subsystem/2(Ref)
  is_ab/1 -> Subsystem/3(FB)
  Alpha-Beta-Zero to abc/1 -> vs*/1

== system B2B_MMC/SM_MMC/MMC2/Control Box MMC2/Insertion Indices (Direct Voltage Control)/Subsystem ==
  Gain1 : Gain  Gain=0.5
  Gain2 : Gain  Gain=m
  Product1 : Product
  Sine Wave1 : Sin  Frequency=w  Phase=[0 2*pi/3 -2*pi/3]  SampleTime=0
  vd1 : Constant  Value=vd_ref
  vs_ref : Outport
  wires:
  vd1/1 -> Gain1/1
  Product1/1 -> vs_ref/1
  Gain1/1 -> Gain2/1
  Gain2/1 -> Product1/1
  Sine Wave1/1 -> Product1/2

== system B2B_MMC/SM_MMC/MMC2/Control Box MMC2/PLL/Subsystem1 ==
  alpha_beta : Inport
  p : Inport  Port=2
  Demux : Demux  Outputs=2
  Gain : Gain
  Product{1..4} (4 alike) : Product
  Sum : Sum  Inputs=|++
  Sum1 : Sum  Inputs=|-+
  Trigonometric Function : Trigonometry  Operator=cos
  Trigonometric Function1 : Trigonometry
  vpcc_d : Outport
  vpcc_q : Outport  Port=2
  wires:
  Trigonometric Function/1 -> Product4/2, Product3/2
  Demux/1 -> Product2/2, Product3/1
  Demux/2 -> Product4/1, Product1/1
  Trigonometric Function1/1 -> Product2/1, Product1/2
  Product1/1 -> Sum/2
  Product2/1 -> Sum1/1
  Product3/1 -> Sum/1
  Product4/1 -> Sum1/2
  alpha_beta/1 -> Demux/1
  p/1 -> Gain/1
  Gain/1 -> Trigonometric Function1/1, Trigonometric Function/1
  Sum1/1 -> vpcc_q/1
  Sum/1 -> vpcc_d/1

== system B2B_MMC/SM_MMC/MMC2/Control Box MMC2/is_ref/dc link voltage control ==
  antiwp : Inport
  vd : Inport  Port=2
  Add : Sum  Inputs=-+
  Add1 : Sum
  Add2 : Sum
  Constant1 : Constant  Value=vd_ref^2
  Divide2 : Product  Inputs=**
  Gain1 : Gain  Gain=cvdc.alpha_id
  Gain2 : Gain  Gain=cvdc.alpha_d*0.5*(Cd+((2*3*Csm)/N))
  Gain3 : Gain  Gain=1/(cvdc.alpha_d*0.5*(Cd+((2*3*Csm)/N)))
  Integrator : Integrator
  filter : TransferFcn  Numerator=[pll.alpha_b*pll.alpha_b]  Denominator=[1 sqrt(2)*pll.alpha_b pll.alpha_b*pll.alpha_b]
  p* : Outport
  wires:
  vd/1 -> filter/1
  filter/1 -> Divide2/2, Divide2/1
  Constant1/1 -> Add/1
  Gain2/1 -> Add2/1, Add1/1
  Add/1 -> Gain2/1
  Divide2/1 -> Add/2
  Add1/1 -> Integrator/1
  Integrator/1 -> Gain1/1
  antiwp/1 -> Gain3/1
  Gain1/1 -> Add2/2
  Add2/1 -> p*/1
  Gain3/1 -> Add1/2

== system B2B_MMC/SM_MMC/MMC1/Control Box MMC1/Controllers/Circulating Current and Arm Energy Controller/BW ==
  note: Butterworth second order LPF alpha_b^2/(s^2+sqrt(2)alpha_b*s+alpha_b^2) implemented with SOGIs kw^2/(s^2+kws+w^2) with k=sqrt(2), w=alpha_b,
  In : Inport
  alpha : Inport  Port=2
  RST : Inport  Port=3
  Divide3 : Product  Inputs=**
  Divide4 : Product  Inputs=**
  Gain7 : Gain  Gain=sqrt(2)
  Gain8 : Gain  Gain=1/sqrt(2)
  Integrator : Integrator  ExternalReset=level
  Integrator1 : Integrator  ExternalReset=level
  Sum1 : Sum  Inputs=-+|
  Sum2 : Sum  Inputs=|+-
  Out : Outport
  wires:
  RST/1 -> Integrator1/2, Integrator/2
  Integrator/1 -> Sum1/1, Integrator1/1
  Integrator1/1 -> Divide4/2
  In/1 -> Sum1/2
  Sum1/1 -> Gain7/1
  alpha/1 -> Divide4/1, Divide3/2
  Divide4/1 -> Gain8/1, Sum2/2
  Divide3/1 -> Integrator/1
  Gain7/1 -> Sum2/1
  Gain8/1 -> Out/1
  Sum2/1 -> Divide3/1

== system B2B_MMC/SM_MMC/MMC1/Control Box MMC1/Controllers/Circulating Current and Arm Energy Controller/arm energy controller  ==
  Divide1 : Product  Inputs=**
  Enable W controller Time: time_enable_W_ctrl : Step  Time=aec.time_enable_W_ctrl  After=aec.enable_W_ctrl  SampleTime=0
  Scope3 : Scope
  Scope7 : Scope
  Scope8 : Scope
  Sum2 : Sum  Inputs=|+-
  Wdelta  Controller : Subsystem
  Wsum  Controller : Subsystem
  delta_i_a : Outport
  wires:
  Sum2/1 -> Divide1/1
  Divide1/1 -> delta_i_a/1, Scope3/1
  Enable W controller Time: time_enable_W_ctrl/1 -> Divide1/2
  Wsum  Controller/1(icWsum*) -> Scope7/1, Sum2/1
  Wdelta  Controller/1(icWdelta*) -> Scope8/1, Sum2/2
  [theta] -> Wdelta  Controller/1(theta)

== system B2B_MMC/SM_MMC/MMC1/Control Box MMC1/Controllers/Circulating Current and Arm Energy Controller/ic controller ==
  ic* : Inport
  Add1 : Sum  Inputs=++++
  Constant2 : Constant  Value=w  SampleTime=-1
  Constant3 : Constant  Value=2*w  SampleTime=-1
  Gain2 : Gain  Gain=ccc.K0
  Gain3 : Gain  Gain=ccc.K1
  Gain4 : Gain  Gain=ccc.K2
  Gain7 : Gain  Gain=ccc.Ra
  Gain8 : Gain  Gain=R
  Integrator : Integrator  ExternalReset=level
  Logical Operator : Logic  Operator=NOT  AllPortsSameDT=off  OutDataTypeStr=boolean
  SOGI1 : Subsystem
  SOGI2 : Subsystem
  Sum4 : Sum  Inputs=--|
  "vc* " : Outport
  wires:
  Logical Operator/1 -> SOGI1/3(RST), Integrator/2
  [enable_W_ctrl2] -> Logical Operator/1
  Gain2/1 -> Add1/4
  Integrator/1 -> Gain2/1
  SOGI2/1(Out) -> Gain4/1
  Sum4/1 -> "vc* "/1
  Constant3/1 -> SOGI2/2(wo)
  Gain4/1 -> Add1/2
  Constant2/1 -> SOGI1/2(wo)
  [IC_RST2] -> SOGI2/3(RST)
  SOGI1/1(Out) -> Gain3/1
  Add1/1 -> Gain7/1
  Gain3/1 -> Add1/3
  ic*/1 -> SOGI1/1(In), Integrator/1, SOGI2/1(In), Add1/1, Gain8/1
  Gain8/1 -> Sum4/1
  Gain7/1 -> Sum4/2

== system B2B_MMC/SM_MMC/MMC1/Control Box MMC1/Controllers/PR Output Current Controller/Subsystem ==
  FF : Inport
  Ref : Inport  Port=2
  FB : Inport  Port=3
  Add : Sum  Inputs=+++
  Constant : Constant  Value=w
  Gain1 : Gain  Gain=occ.Kp
  Gain2 : Gain  Gain=1/occ.Kp
  Modulation : Scope
  Mux1 : Mux  Inputs=2
  PR : Subsystem
  Saturation : Saturate  UpperLimit=vsp_max  LowerLimit=-vsp_max
  Sum : Sum  Inputs=|+-
  Sum1 : Sum  Inputs=|++
  Sum2 : Sum  Inputs=-+|
  vsAB_ref : Outport
  wires:
  Sum1/1 -> PR/1(In)
  Gain2/1 -> Sum1/2
  Sum/1 -> Sum1/1, Gain1/1
  PR/1(Out) -> Add/3
  Ref/1 -> Mux1/1, Sum/1
  Sum2/1 -> Gain2/1
  Gain1/1 -> Add/2
  Constant/1 -> PR/2(w0)
  Add/1 -> Saturation/1, Sum2/1
  FB/1 -> Sum/2, Mux1/2
  FF/1 -> Add/1
  Mux1/1 -> Modulation/1
  Saturation/1 -> vsAB_ref/1, Sum2/2

== system B2B_MMC/SM_MMC/MMC2/Control Box MMC2/Controllers/Circulating Current and Arm Energy Controller/BW ==
  note: Butterworth second order LPF alpha_b^2/(s^2+sqrt(2)alpha_b*s+alpha_b^2) implemented with SOGIs kw^2/(s^2+kws+w^2) with k=sqrt(2), w=alpha_b,
  In : Inport
  alpha : Inport  Port=2
  RST : Inport  Port=3
  Divide3 : Product  Inputs=**
  Divide4 : Product  Inputs=**
  Gain7 : Gain  Gain=sqrt(2)
  Gain8 : Gain  Gain=1/sqrt(2)
  Integrator : Integrator  ExternalReset=level
  Integrator1 : Integrator  ExternalReset=level
  Sum1 : Sum  Inputs=-+|
  Sum2 : Sum  Inputs=|+-
  Out : Outport
  wires:
  RST/1 -> Integrator1/2, Integrator/2
  Integrator/1 -> Sum1/1, Integrator1/1
  Integrator1/1 -> Divide4/2
  In/1 -> Sum1/2
  Sum1/1 -> Gain7/1
  alpha/1 -> Divide4/1, Divide3/2
  Divide4/1 -> Gain8/1, Sum2/2
  Divide3/1 -> Integrator/1
  Gain7/1 -> Sum2/1
  Gain8/1 -> Out/1
  Sum2/1 -> Divide3/1

== system B2B_MMC/SM_MMC/MMC2/Control Box MMC2/Controllers/Circulating Current and Arm Energy Controller/arm energy controller  ==
  Divide1 : Product  Inputs=**
  Enable W controller Time: time_enable_W_ctrl : Step  Time=aec.time_enable_W_ctrl  After=aec.enable_W_ctrl  SampleTime=0
  Scope3 : Scope
  Scope7 : Scope
  Scope8 : Scope
  Sum2 : Sum  Inputs=|+-
  Wdelta  Controller : Subsystem
  Wsum  Controller : Subsystem
  delta_i_a : Outport
  wires:
  Sum2/1 -> Divide1/1
  Divide1/1 -> delta_i_a/1, Scope3/1
  Enable W controller Time: time_enable_W_ctrl/1 -> Divide1/2
  Wsum  Controller/1(icWsum*) -> Scope7/1, Sum2/1
  Wdelta  Controller/1(icWdelta*) -> Scope8/1, Sum2/2
  [theta] -> Wdelta  Controller/1(theta)

== system B2B_MMC/SM_MMC/MMC2/Control Box MMC2/Controllers/Circulating Current and Arm Energy Controller/ic controller ==
  ic* : Inport
  Add1 : Sum  Inputs=++++
  Constant2 : Constant  Value=w  SampleTime=-1
  Constant3 : Constant  Value=2*w  SampleTime=-1
  Gain2 : Gain  Gain=ccc.K0
  Gain3 : Gain  Gain=ccc.K1
  Gain4 : Gain  Gain=ccc.K2
  Gain7 : Gain  Gain=ccc.Ra
  Gain8 : Gain  Gain=R
  Integrator : Integrator  ExternalReset=level
  Logical Operator : Logic  Operator=NOT  AllPortsSameDT=off  OutDataTypeStr=boolean
  SOGI1 : Subsystem
  SOGI2 : Subsystem
  Sum4 : Sum  Inputs=--|
  "vc* " : Outport
  wires:
  Logical Operator/1 -> SOGI1/3(RST), Integrator/2
  [enable_W_ctrl2] -> Logical Operator/1
  Gain2/1 -> Add1/4
  Integrator/1 -> Gain2/1
  SOGI2/1(Out) -> Gain4/1
  Sum4/1 -> "vc* "/1
  Constant3/1 -> SOGI2/2(wo)
  Gain4/1 -> Add1/2
  Constant2/1 -> SOGI1/2(wo)
  [IC_RST2] -> SOGI2/3(RST)
  SOGI1/1(Out) -> Gain3/1
  Add1/1 -> Gain7/1
  Gain3/1 -> Add1/3
  ic*/1 -> SOGI1/1(In), Integrator/1, SOGI2/1(In), Add1/1, Gain8/1
  Gain8/1 -> Sum4/1
  Gain7/1 -> Sum4/2

== system B2B_MMC/SM_MMC/MMC2/Control Box MMC2/Controllers/PR Output Current Controller/Subsystem ==
  FF : Inport
  Ref : Inport  Port=2
  FB : Inport  Port=3
  Add : Sum  Inputs=+++
  Constant : Constant  Value=w
  Gain1 : Gain  Gain=occ.Kp
  Gain2 : Gain  Gain=1/occ.Kp
  Modulation : Scope
  Mux1 : Mux  Inputs=2
  PR : Subsystem
  Saturation : Saturate  UpperLimit=vsp_max  LowerLimit=-vsp_max
  Sum : Sum  Inputs=|+-
  Sum1 : Sum  Inputs=|++
  Sum2 : Sum  Inputs=-+|
  vsAB_ref : Outport
  wires:
  Sum1/1 -> PR/1(In)
  Gain2/1 -> Sum1/2
  Sum/1 -> Sum1/1, Gain1/1
  PR/1(Out) -> Add/3
  Ref/1 -> Mux1/1, Sum/1
  Sum2/1 -> Gain2/1
  Gain1/1 -> Add/2
  Constant/1 -> PR/2(w0)
  Add/1 -> Saturation/1, Sum2/1
  FB/1 -> Sum/2, Mux1/2
  FF/1 -> Add/1
  Mux1/1 -> Modulation/1
  Saturation/1 -> vsAB_ref/1, Sum2/2

== system B2B_MMC/SM_MMC/MMC1/Control Box MMC1/Controllers/Circulating Current and Arm Energy Controller/arm energy controller /Wdelta  Controller ==
  theta : Inport
  "  Wdelta*" : Constant  Value=0
  Demux2 : Demux  Outputs=3
  Goto Tag Visibility : GotoTagVisibility  GotoTag=ca
  Goto Tag Visibility1 : GotoTagVisibility  GotoTag=cb
  Goto Tag Visibility2 : GotoTagVisibility  GotoTag=cc
  Kp_Wdelta : Gain  Gain=aec.Kp_Wdelta
  Mux : Mux  Inputs=2
  Mux1 : Mux  Inputs=3
  Scope7 : Scope
  Sum6 : Sum  Inputs=+-
  correction : Subsystem
  ripple pass (leg a) : Subsystem
  ripple pass (leg b) : Subsystem
  ripple pass (leg c) : Subsystem
  icWdelta* : Outport
  tag scope: ca=scoped, cb=scoped, cc=scoped
  wires:
  "  Wdelta*"/1 -> Sum6/1, Mux/1
  Sum6/1 -> Kp_Wdelta/1
  Mux1/1 -> Mux/2, Sum6/2
  Mux/1 -> Scope7/1
  ripple pass (leg a)/1(Out1) -> Mux1/1
  ripple pass (leg b)/1(Out1) -> Mux1/2
  ripple pass (leg c)/1(Out1) -> Mux1/3
  Kp_Wdelta/1 -> Demux2/1
  Demux2/1 -> [ca]
  Demux2/2 -> [cb]
  Demux2/3 -> [cc]
  theta/1 -> correction/1(theta)
  correction/1(delta_i) -> icWdelta*/1
  [vc_la] -> ripple pass (leg a)/2(vc_la)
  [vc_ua] -> ripple pass (leg a)/1(vc_ua)
  [vc_ub] -> ripple pass (leg b)/1(vc_ub)
  [vc_lb] -> ripple pass (leg b)/2(vc_lb)
  [vc_uc] -> ripple pass (leg c)/1(vc_uc)
  [vc_lc] -> ripple pass (leg c)/2(vc_lc)

== system B2B_MMC/SM_MMC/MMC1/Control Box MMC1/Controllers/Circulating Current and Arm Energy Controller/arm energy controller /Wsum  Controller ==
  Kp_Wsum : Gain  Gain=aec.Kp_Wsum
  Mux : Mux  Inputs=2
  Mux1 : Mux  Inputs=3
  Product1 : Product
  Ripple Pass (leg a) : Subsystem
  Ripple Pass (leg b) : Subsystem
  Ripple Pass (leg c) : Subsystem
  Scope7 : Scope
  Step : Step  Time=aec.time_WsumRef_step  Before=1  After=1+aec.WsumRefStep*aec.enable_Wsum_step  SampleTime=0
  Sum6 : Sum  Inputs=+-
  "Wsum* " : Constant  Value=WsumRef
  icWsum* : Outport
  wires:
  Mux1/1 -> Sum6/2, Mux/2
  Sum6/1 -> Kp_Wsum/1
  Step/1 -> Product1/2
  Product1/1 -> Mux/1, Sum6/1
  "Wsum* "/1 -> Product1/1
  Kp_Wsum/1 -> icWsum*/1
  Mux/1 -> Scope7/1
  Ripple Pass (leg b)/1(Out1) -> Mux1/2
  Ripple Pass (leg a)/1(Out1) -> Mux1/1
  Ripple Pass (leg c)/1(Out1) -> Mux1/3
  [vc_ua] -> Ripple Pass (leg a)/1(vc_ua)
  [vc_la] -> Ripple Pass (leg a)/2(vc_la)
  [vc_lb] -> Ripple Pass (leg b)/2(vc_lb)
  [vc_ub] -> Ripple Pass (leg b)/1(vc_ub)
  [vc_lc] -> Ripple Pass (leg c)/2(vc_lc)
  [vc_uc] -> Ripple Pass (leg c)/1(vc_uc)

== system B2B_MMC/SM_MMC/MMC1/Control Box MMC1/Controllers/Circulating Current and Arm Energy Controller/ic controller/SOGI1 ==
  In : Inport
  wo : Inport  Port=2
  RST : Inport  Port=3
  Divide : Product  Inputs=**
  Divide1 : Product  Inputs=**
  Divide2 : Product  Inputs=*/
  Integrator : Integrator  ExternalReset=level
  Integrator1 : Integrator  ExternalReset=level
  Sum3 : Sum  Inputs=|+-
  Out : Outport
  wires:
  Divide1/1 -> Sum3/2
  Divide/1 -> Integrator/1
  Sum3/1 -> Divide/1
  Integrator1/1 -> Divide1/2
  In/1 -> Sum3/1
  Divide2/1 -> Out/1
  RST/1 -> Integrator/2, Integrator1/2
  wo/1 -> Divide2/2, Divide1/1, Divide/2
  Integrator/1 -> Divide2/1, Integrator1/1

== system B2B_MMC/SM_MMC/MMC1/Control Box MMC1/Controllers/Circulating Current and Arm Energy Controller/ic controller/SOGI2 ==
  In : Inport
  wo : Inport  Port=2
  RST : Inport  Port=3
  Divide : Product  Inputs=**
  Divide1 : Product  Inputs=**
  Divide2 : Product  Inputs=*/
  Integrator : Integrator  ExternalReset=level  LimitOutput=on  UpperSaturationLimit=is_max  LowerSaturationLimit=-is_max
  Integrator1 : Integrator  ExternalReset=level  LimitOutput=on  UpperSaturationLimit=is_max  LowerSaturationLimit=-is_max
  Sum3 : Sum  Inputs=|+-
  Out : Outport
  wires:
  Integrator/1 -> Divide2/1, Integrator1/1
  wo/1 -> Divide/2, Divide1/1, Divide2/2
  RST/1 -> Integrator/2, Integrator1/2
  Divide2/1 -> Out/1
  In/1 -> Sum3/1
  Integrator1/1 -> Divide1/2
  Sum3/1 -> Divide/1
  Divide/1 -> Integrator/1
  Divide1/1 -> Sum3/2

== system B2B_MMC/SM_MMC/MMC1/Control Box MMC1/Controllers/PR Output Current Controller/Subsystem/PR ==
  note: SOGI continuous=sw/(s2+w2)
  In : Inport
  w0 : Inport  Port=2
  Gain3 : Gain  Gain=occ.K1
  SOGI : Subsystem
  Step : Step  Time=0.0001  Before=1  After=0  SampleTime=0
  Out : Outport
  wires:
  Gain3/1 -> Out/1
  In/1 -> SOGI/1(In)
  w0/1 -> SOGI/2(wo)
  [occRST] -> SOGI/3(RST)
  SOGI/1(Out) -> Gain3/1
  Step/1 -> [occRST]

== system B2B_MMC/SM_MMC/MMC2/Control Box MMC2/Controllers/Circulating Current and Arm Energy Controller/arm energy controller /Wdelta  Controller ==
  theta : Inport
  "  Wdelta*" : Constant  Value=0
  Demux2 : Demux  Outputs=3
  Goto Tag Visibility : GotoTagVisibility  GotoTag=ca
  Goto Tag Visibility1 : GotoTagVisibility  GotoTag=cb
  Goto Tag Visibility2 : GotoTagVisibility  GotoTag=cc
  Kp_Wdelta : Gain  Gain=aec.Kp_Wdelta
  Mux : Mux  Inputs=2
  Mux1 : Mux  Inputs=3
  Scope7 : Scope
  Sum6 : Sum  Inputs=+-
  correction : Subsystem
  ripple pass (leg a) : Subsystem
  ripple pass (leg b) : Subsystem
  ripple pass (leg c) : Subsystem
  icWdelta* : Outport
  tag scope: ca=scoped, cb=scoped, cc=scoped
  wires:
  "  Wdelta*"/1 -> Sum6/1, Mux/1
  Sum6/1 -> Kp_Wdelta/1
  Mux1/1 -> Mux/2, Sum6/2
  Mux/1 -> Scope7/1
  ripple pass (leg a)/1(Out1) -> Mux1/1
  ripple pass (leg b)/1(Out1) -> Mux1/2
  ripple pass (leg c)/1(Out1) -> Mux1/3
  Kp_Wdelta/1 -> Demux2/1
  Demux2/1 -> [ca]
  Demux2/2 -> [cb]
  Demux2/3 -> [cc]
  theta/1 -> correction/1(theta)
  correction/1(delta_i) -> icWdelta*/1
  [vc_la] -> ripple pass (leg a)/2(vc_la)
  [vc_ua] -> ripple pass (leg a)/1(vc_ua)
  [vc_ub] -> ripple pass (leg b)/1(vc_ub)
  [vc_lb] -> ripple pass (leg b)/2(vc_lb)
  [vc_uc] -> ripple pass (leg c)/1(vc_uc)
  [vc_lc] -> ripple pass (leg c)/2(vc_lc)
